simulink model "Env_Agent_Simulation"  (R2024a)
settings: Solver=VariableStepAuto  StartTime=0.0  StopTime=10.0  RelTol=1e-3
libraries: simulink x2, embmathops x1, rllib x1
settings Model: Creator=sameb  LastModifiedBy=sameb
settings ModelReferenceCC: ModelReferenceMinAlgLoopOccurrences=on

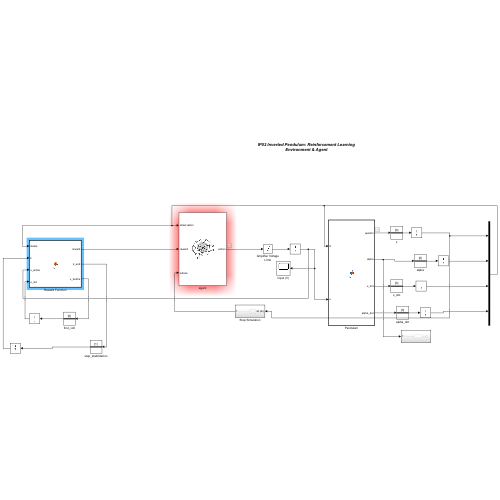
[thumbnail: Simulink's stored preview of the top-level diagram]
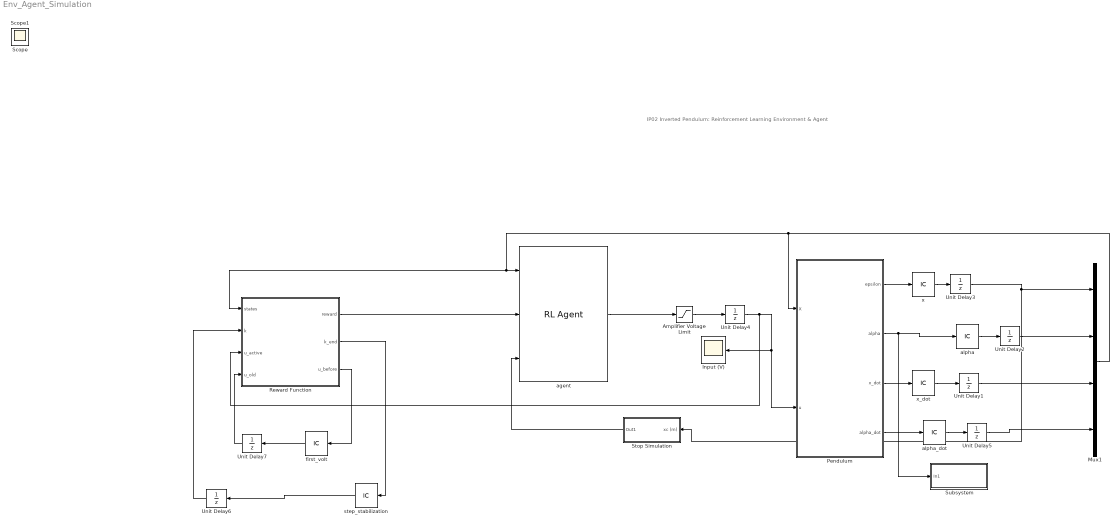
== system Env_Agent_Simulation ==
  note: IP02 Inverted Pendulum: Reinforcement Learning Environment & Agent
  Amplifier Voltage Limit : Saturate  UpperLimit=10  LowerLimit=-10
  Input (V) : Scope
  Mux1 : Mux
  Pendulum : MATLAB Function  TreatAsAtomicUnit=on
  Reward Function : MATLAB Function  TreatAsAtomicUnit=on
  Stop Simulation : Subsystem
  Subsystem : Subsystem
  Unit Delay{1..7} (7 alike) : UnitDelay  SampleTime=-1  HasFrameUpgradeWarning=on
  agent : rllib/RL Agent  Agent=agent  ExternalActionAsInput=off  ProvideLastAction=off  ProvideCumRwd=off  TreatAsDirectFeedthrough=on  UseStrictObservationDataTypes=off
      link override external action: Value=0
  alpha : InitialCondition  Value=0
  alpha_dot : InitialCondition  Value=0
  first_volt : InitialCondition  Value=0
  step_stabilization : InitialCondition
  x : InitialCondition  Value=0
  x_dot : InitialCondition  Value=0
  Scope : Scope
  Scope1 : Scope
  wires:
  Reward Function/1(reward) -> agent/2
  Stop Simulation/1(Out1) -> agent/3
  agent/1 -> Amplifier Voltage Limit/1
  Pendulum/4(alpha_dot) -> alpha_dot/1
  Pendulum/1(epsilon) -> x/1
  Pendulum/2(alpha) -> Subsystem/1(In1), alpha/1
  Pendulum/3(x_dot) -> x_dot/1
  Mux1/1 -> agent/1, Reward Function/1(states), Pendulum/1(X)
  Amplifier Voltage Limit/1 -> Unit Delay4/1
  Unit Delay4/1 -> Reward Function/3(u_active), Input (V)/1, Pendulum/2(u)
  x/1 -> Unit Delay3/1
  alpha/1 -> Unit Delay2/1
  Unit Delay2/1 -> Mux1/2
  Unit Delay3/1 -> Mux1/1, Stop Simulation/1(xc (m))
  x_dot/1 -> Unit Delay1/1
  Unit Delay1/1 -> Mux1/3
  alpha_dot/1 -> Unit Delay5/1
  Unit Delay5/1 -> Mux1/4
  Reward Function/2(k_end) -> step_stabilization/1
  step_stabilization/1 -> Unit Delay6/1
  Unit Delay6/1 -> Reward Function/2(k)
  Unit Delay7/1 -> Reward Function/4(u_old)
  Reward Function/3(u_before) -> first_volt/1
  first_volt/1 -> Unit Delay7/1

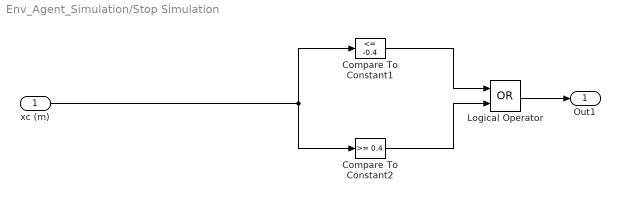
== system Env_Agent_Simulation/Stop Simulation ==
  xc (m) : Inport
  Compare To Constant1 : simulink/Logic and Bit Operations/Compare To Constant  relop=<=  const=-0.4  OutDataTypeStr=boolean
  Compare To Constant2 : simulink/Logic and Bit Operations/Compare To Constant  relop=>=  const=0.4  OutDataTypeStr=boolean
  Logical Operator : Logic  Operator=OR  AllPortsSameDT=off  OutDataTypeStr=boolean
  Out1 : Outport
  wires:
  Logical Operator/1 -> Out1/1
  Compare To Constant2/1 -> Logical Operator/2
  Compare To Constant1/1 -> Logical Operator/1
  xc (m)/1 -> Compare To Constant1/1, Compare To Constant2/1

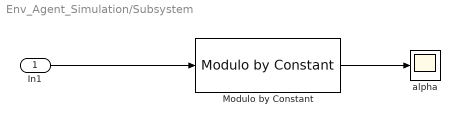
== system Env_Agent_Simulation/Subsystem ==
  In1 : Inport
  Modulo by Constant : embmathops/Modulo by Constant  Denominator=2 * pi  SimulateUsing=Code generation
      settings: LibrarySourceBlock=embeddedMathLib/Modulo by Constant
  alpha : Scope
  wires:
  In1/1 -> Modulo by Constant/1
  Modulo by Constant/1 -> alpha/1

== matlab function Env_Agent_Simulation/Pendulum ==
  data: X input double size=[4 1]; u input double size=[1 1]; epsilon output double size=[1 1]; alpha output double size=[1 1]; x_dot output double size=[1 1]; alpha_dot output double size=[1 1]
function [epsilon, alpha,x_dot,alpha_dot]= fcn(X, u)

[epsilon, alpha,x_dot,alpha_dot] = DynamicPendulum(X,u);

== matlab function Env_Agent_Simulation/Reward Function ==
  data: states input double size=[4 1]; reward output double size=[1 1]; k input double size=[1 1]; k_end output double size=[1 1]; u_active input double size=[1 1]; u_old input double size=[1 1]; u_before output double size=[1 1]
function [reward,k_end, u_before] = fcn(states,k, u_active, u_old)
[reward,k_end]=RewardPendulum(states,k, u_active, u_old);
u_before = u_active;
end
